simulink model "SimuLink_Testing_Model"  (R2024a)
settings: Solver=ode4  StartTime=0.0  StopTime=10.0  FixedStep=0.001  RelTol=1e-3
undefined symbols (not defined in the file): initial_position, initial_velocity, mass, spring_constant
settings Model: Creator=641893  LastModifiedBy=641893

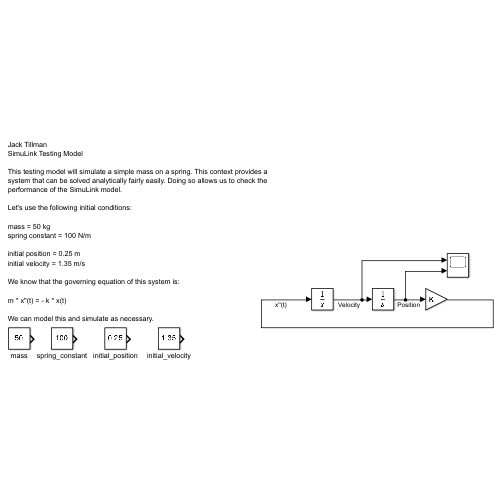
[thumbnail: Simulink's stored preview of the top-level diagram]
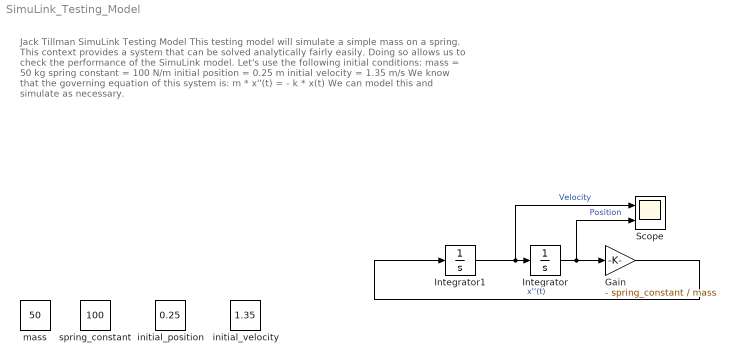
== system SimuLink_Testing_Model ==
  note: Jack Tillman
      | SimuLink Testing Model
      |
      | This testing model will simulate a simple mass on a spring. This context provides a system that can be solved analytically fairly easily. Doing so allows us to check the performance of the SimuLink model.
      |
      | Let's use the following initial conditions:
      |
      | mass = 50 kg
      | spring constant = 100 N/m
      |
      | initial position = 0.25 m
      | initial velocity = 1.35 m/s
      |
      | We know that the governing equation of this system is:
      |
      | m * x''(t) = - k * x(t)
      |
      | We can model this and simulate as necessary.
  Gain : Gain  Gain=- spring_constant / mass
  Integrator : Integrator  InitialCondition=initial_position
  Integrator1 : Integrator  InitialCondition=initial_velocity
  Scope : Scope  NumInputPorts=2
  initial_position : Constant  Value=0.25
  initial_velocity : Constant  Value=1.35
  mass : Constant  Value=50
  spring_constant : Constant  Value=100
  wires:
  Integrator1/1 -> Scope/1, Integrator/1  "Velocity"
  Gain/1 -> Integrator1/1  "x''(t)"
  Integrator/1 -> Scope/2, Gain/1  "Position"
